simulink model "Tim1"  (R2019b)
settings: Solver=VariableStepAuto  StartTime=0.0  StopTime=10.0  RelTol=1e-3
undefined symbols (not defined in the file): A, B, ContractAssumeBlock, ContractBlock, ContractGuaranteeBlock, ContractValidatorBlock
libraries: cocosimLibs x1
settings Model: Creator=hbourbou  LastModifiedBy=hbourbou

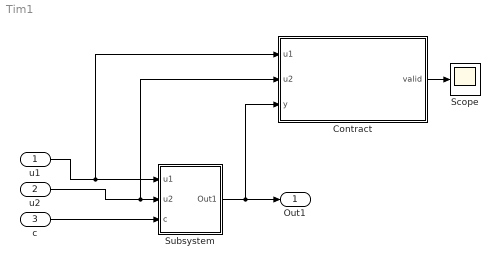
== system Tim1 ==
  u1 : Inport
  u2 : Inport  Port=2
  c : Inport  Port=3
  Contract : Subsystem  mask(ContractBlock){ContractBlockType=ContractBlock, ShowInLibBrowser=on}
      mask init:
      | set_param(gcb, 'LinkStatus', 'none');
      settings: CopyFcn=set_param(gcb, 'LinkStatus', 'none');
      mask DialogControl DescTextVar Prompt: Contract block
      mask Display: text(0.5, 0.5, '{\bf\fontsize{20}Contract}', 'hor', 'center', 'texmode','on');
  Scope : Scope
  Subsystem : Subsystem
  Out1 : Outport
  wires:
  u1/1 -> Contract/1(u1), Subsystem/1(u1)
  u2/1 -> Contract/2(u2), Subsystem/2(u2)
  c/1 -> Subsystem/3(c)
  Subsystem/1(Out1) -> Contract/3(y), Out1/1
  Contract/1(valid) -> Scope/1

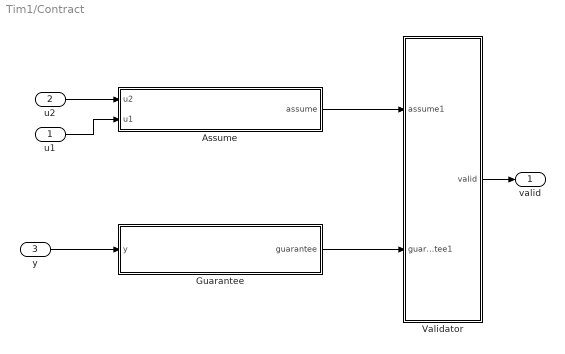
== system Tim1/Contract ==
  u1 : Inport
  u2 : Inport  Port=2
  y : Inport  Port=3
  Assume : Subsystem  mask(ContractAssumeBlock){ContractBlockType=ContractAssumeBlock}
      mask init:
      | set_param(gcb, 'LinkStatus', 'none');
      mask DialogControl DescTextVar Prompt: Assume block
      mask Display: text(0.5, 0.5, '{\bf\fontsize{20}Assume}', 'hor', 'center', 'texmode','on');
  Guarantee : Subsystem  mask(ContractGuaranteeBlock){ContractBlockType=ContractGuaranteeBlock}
      mask init:
      | set_param(gcb, 'LinkStatus', 'none');
      mask DialogControl DescTextVar Prompt: Guarantee block
      mask Display: text(0.5, 0.5, '{\bf\fontsize{20}Guarantee}', 'hor', 'center', 'texmode','on');
  Validator : Subsystem  mask(ContractValidatorBlock){assumePorts=1, guaranteePorts=1, modePorts=0, ContractBlockType=ContractValidatorBlock}
      mask prompts: assumePorts "Assume ports     :"; guaranteePorts "Guarantee ports :"; modePorts "Mode ports        :"
      mask help: The validator block implements the following logic: <br> <br> <b>Sofar</b>(assume<sub>1</sub> <b>&#8743;</b> assume<sub>2</sub> <b>&#8743;</b> ... assume<sub>k</sub>) <b>&rarr;</b> <b>Sofar</b>(guarantee<sub>1</sub> <b>&#8743;</b> guarantee<sub>2</sub> <b>&#8743;</b> ... guarantee<sub>m</sub> <b>&#8743;</b> mode<sub>1</sub> <b>&#8743;</b> mode<sub>2</sub> <b>&#8743;</b> ... <b>&#8743;</b> mode<sub>n</sub> )<br> where mode<sub>i</sub> = require<sub>i</sub> <b>&rarr;</b> ensure<sub>i</sub>
      mask init:
      | set_param(gcb,'LinkStatus','none');
      | coco_blockCallbacks.CoCoSimContract.validatorCallback(gcb);
      mask Display: disp(' ')
  valid : Outport
  wires:
  Validator/1(valid) -> valid/1
  Assume/1(assume) -> Validator/1(assume1)
  Guarantee/1(guarantee) -> Validator/2(guarantee1)
  y/1 -> Guarantee/1(y)
  u2/1 -> Assume/1(u2)
  u1/1 -> Assume/2(u1)

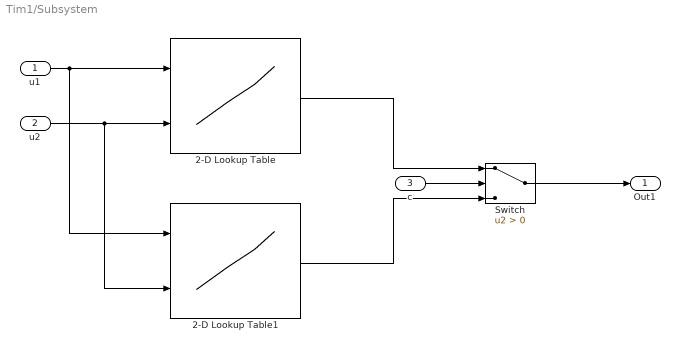
== system Tim1/Subsystem ==
  u1 : Inport
  u2 : Inport  Port=2
  c : Inport  Port=3
  2-D Lookup Table : Lookup_n-D  BreakpointsForDimension1=[0, 5000, 10000, 15000, 20000, 30000]  BreakpointsForDimension2=[135; 200; 245; 250; 270]  Table=B  ExtrapMethod=Clip  InternalRulePriority=Speed  RndMeth=Simplest  InputSameDT=on
  2-D Lookup Table1 : Lookup_n-D  BreakpointsForDimension1=[0, 5000, 10000, 15000, 20000, 30000]  BreakpointsForDimension2=[135; 200; 245; 250; 270]  Table=A  ExtrapMethod=Clip  InternalRulePriority=Speed  RndMeth=Simplest  InputSameDT=on
  Switch : Switch  Criteria=u2 > Threshold
  Out1 : Outport
  wires:
  Switch/1 -> Out1/1
  2-D Lookup Table1/1 -> Switch/3
  c/1 -> Switch/2
  u2/1 -> 2-D Lookup Table1/2, 2-D Lookup Table/2
  u1/1 -> 2-D Lookup Table1/1, 2-D Lookup Table/1
  2-D Lookup Table/1 -> Switch/1

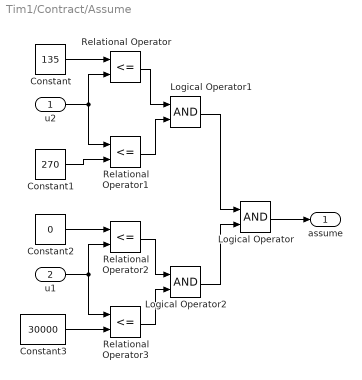
== system Tim1/Contract/Assume ==
  u2 : Inport
  u1 : Inport  Port=2
  Constant : Constant  Value=135
  Constant1 : Constant  Value=270
  Constant2 : Constant  Value=0
  Constant3 : Constant  Value=30000
  Logical Operator : Logic  AllPortsSameDT=off  OutDataTypeStr=boolean
  Logical Operator1 : Logic  AllPortsSameDT=off  OutDataTypeStr=boolean
  Logical Operator2 : Logic  AllPortsSameDT=off  OutDataTypeStr=boolean
  Relational Operator{,1..3} (4 alike) : RelationalOperator  Operator=<=  OutDataTypeStr=boolean  RndMeth=Simplest
  assume : Outport  OutDataTypeStr=boolean
  wires:
  Logical Operator/1 -> assume/1
  Logical Operator1/1 -> Logical Operator/1
  Logical Operator2/1 -> Logical Operator/2
  Constant/1 -> Relational Operator/1
  u2/1 -> Relational Operator/2, Relational Operator1/1
  Relational Operator/1 -> Logical Operator1/1
  Relational Operator1/1 -> Logical Operator1/2
  Constant1/1 -> Relational Operator1/2
  Relational Operator2/1 -> Logical Operator2/1
  u1/1 -> Relational Operator2/2, Relational Operator3/1
  Constant3/1 -> Relational Operator3/2
  Relational Operator3/1 -> Logical Operator2/2
  Constant2/1 -> Relational Operator2/1

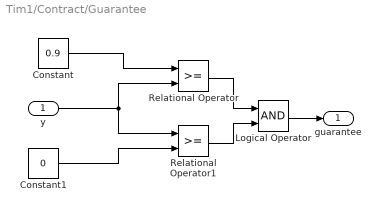
== system Tim1/Contract/Guarantee ==
  y : Inport
  Constant : Constant  Value=0.9
  Constant1 : Constant  Value=0
  Logical Operator : Logic  AllPortsSameDT=off  OutDataTypeStr=boolean
  Relational Operator : RelationalOperator  OutDataTypeStr=boolean  RndMeth=Simplest
  Relational Operator1 : RelationalOperator  OutDataTypeStr=boolean  RndMeth=Simplest
  guarantee : Outport  OutDataTypeStr=boolean
  wires:
  Logical Operator/1 -> guarantee/1
  y/1 -> Relational Operator1/1, Relational Operator/2
  Constant/1 -> Relational Operator/1
  Relational Operator/1 -> Logical Operator/1
  Constant1/1 -> Relational Operator1/2
  Relational Operator1/1 -> Logical Operator/2

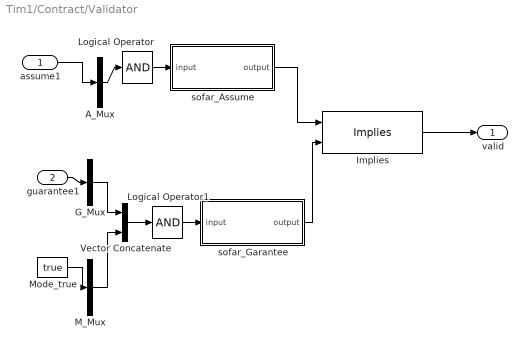
== system Tim1/Contract/Validator ==
  assume1 : Inport  OutDataTypeStr=boolean  PortDimensions=1
  guarantee1 : Inport  Port=2  OutDataTypeStr=boolean  PortDimensions=1
  A_Mux : Mux  Inputs=1
  G_Mux : Mux  Inputs=1
  Implies : cocosimLibs/Implies  SystemSampleTime=-1  Latency=0  AutoFrameSizeCalculation=off
      settings: SourceProductName=CoCoSim Specification Library
  Logical Operator : Logic  Inputs=1  AllPortsSameDT=off  OutDataTypeStr=boolean
  Logical Operator1 : Logic  Inputs=1  AllPortsSameDT=off  OutDataTypeStr=boolean
  M_Mux : Mux  Inputs=1
  Mode_true : Constant  Value=true  OutDataTypeStr=boolean
  Vector Concatenate : Concatenate
  sofar_Assume : Subsystem
  sofar_Garantee : Subsystem
  valid : Outport
  wires:
  sofar_Assume/1(output) -> Implies/1
  sofar_Garantee/1(output) -> Implies/2
  Implies/1 -> valid/1
  A_Mux/1 -> Logical Operator/1
  Logical Operator/1 -> sofar_Assume/1(input)
  Logical Operator1/1 -> sofar_Garantee/1(input)
  G_Mux/1 -> Vector Concatenate/1
  guarantee1/1 -> G_Mux/1
  assume1/1 -> A_Mux/1
  Vector Concatenate/1 -> Logical Operator1/1
  M_Mux/1 -> Vector Concatenate/2
  Mode_true/1 -> M_Mux/1

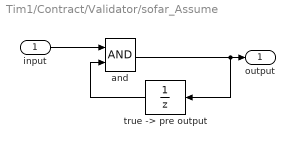
== system Tim1/Contract/Validator/sofar_Assume ==
  input : Inport  OutDataTypeStr=boolean
  and : Logic  AllPortsSameDT=off  OutDataTypeStr=boolean
  "true -> pre output" : UnitDelay  InitialCondition=true  SampleTime=-1  HasFrameUpgradeWarning=on
  output : Outport  OutDataTypeStr=boolean
  wires:
  input/1 -> and/1
  "true -> pre output"/1 -> and/2
  and/1 -> "true -> pre output"/1, output/1

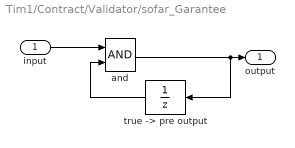
== system Tim1/Contract/Validator/sofar_Garantee ==
  input : Inport  OutDataTypeStr=boolean
  and : Logic  AllPortsSameDT=off  OutDataTypeStr=boolean
  "true -> pre output" : UnitDelay  InitialCondition=true  SampleTime=-1  HasFrameUpgradeWarning=on
  output : Outport  OutDataTypeStr=boolean
  wires:
  input/1 -> and/1
  "true -> pre output"/1 -> and/2
  and/1 -> "true -> pre output"/1, output/1
